simulink model "FPGA_MODELSIM"  (R2019b)
settings: Solver=ode1  StartTime=0.0  StopTime=1  FixedStep=1e-4  RelTol=1e-3
InitFcn:
  | Ts=1e-4
  | T=1e-5
values from neighbouring files (symbols this model uses):
  B = 0.0136    [Pmsm.m]
  J = 0.0027    [Pmsm.m]
  Kiq = double(Kiq)    [Pmsm.m]
  Kiw = double(Kiw)    [Pmsm.m]
  Kpq = double(Kpq)    [Pmsm.m]
  Kpw = double(Kpw)    [Pmsm.m]
  Lambda_m = 0.2026    [Pmsm.m]
  Ld = 19.75e-3    (= 0.01975)    [Pmsm.m]
  Lq = 22.5e-3    (= 0.0225)    [Pmsm.m]
  P = 8    [Pmsm.m]
  Rs = 1.477    [Pmsm.m]
libraries: modelsimlib x2
settings Model: Creator=samfi  LastModifiedBy=samfi

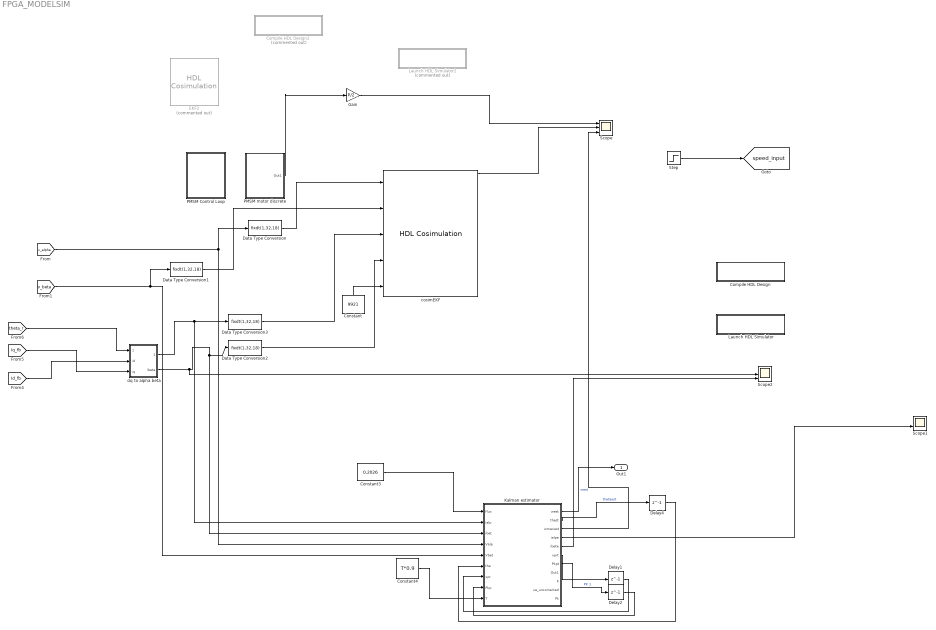
== system FPGA_MODELSIM ==
  Compile HDL Design : Subsystem
      settings: OpenFcn=eval('compile_hdl_design_cosimEKF');
      mask Display: disp(['Double-Click to' char(10) 'compile HDL files'])
  Compile HDL Design2 : Subsystem  Commented=on
      settings: OpenFcn=eval('compile_hdl_design_EKF');
      mask Display: disp(['Double-Click to' char(10) 'compile HDL files'])
  Constant : Constant  Value=9921  OutDataTypeStr=uint32  SampleTime=1e-4
  Constant3 : Constant  Value=0.2026
  Constant4 : Constant  Value=T*0.9  SampleTime=1e-4
  Data Type Conversion{,1..3} (4 alike) : DataTypeConversion  OutDataTypeStr=fixdt(1,32,18)
  Delay1 : Delay  DelayLength=1  InitialCondition=0
  Delay2 : Delay  DelayLength=1  InitialCondition=0
  Delay4 : Delay  DelayLength=1  InitialCondition=0
  EKF2 : modelsimlib/HDL Cosimulation  Commented=on  PortPaths=/EKF/valpha;/EKF/vbeta;/EKF/ialpham;/EKF/ibetam;/EKF/ctheta;/EKF/stheta;/EKF/nbSamples;/EKF/omega;/EKF/theta  PortModes=[1 1 1 1 1 1 1 2 2 ]  PortTimes=[-1,-1,-1,-1,-1,-1,-1,1e-4,1e-4]  PortSigns=[-1 -1 -1 -1 -1 -1 -1 1 1 ]  PortFracLengths=[0,0,0,0,0,0,0,18,18]  CommLocal=on  CommSharedMemory=on  CommPortNumber=4449  CommShowInfo=on  ClockModes=[]  ClockTimes=[]  TclPreSimCommand=|  TclPostSimCommand=|  TimingMode=s  TimingScaleFactor=1  idxCellArray={'UNUSED_VAR'}  CosimBypass=Full Simulation  AllowDirectFeedthrough=on  ProductName=EDA Simulator Link MQ  RunAutoTimescale=off  HdlClocks=/EKF/clk 10 ns;  PreRunTime=10  PreRunTimeUnit=ns
      TclPreSimCommand=|
      | force /EKF/clk 0 0 ns, 1 5 ns -repeat 10 ns;
      | force /EKF/reset 0 0 ns, 1 8 ns;
      TclPostSimCommand=|
      | noforce /EKF/clk;
      | noforce /EKF/reset;
      | puts "done";
      settings: SourceProductName=HDL Verifier  SourceProductBaseCode=ES
  Gain : Gain  Gain=P/2
  Kalman estimator : Subsystem  SystemSampleTime=1e-4
  Launch HDL Simulator : Subsystem
      settings: OpenFcn=eval('launch_hdl_simulator_cosimEKF');
      mask Display: disp(['Double-Click to' char(10) 'launch HDL simulator'])
  Launch HDL Simulator2 : Subsystem  Commented=on
      settings: OpenFcn=eval('launch_hdl_simulator_EKF');
      mask Display: disp(['Double-Click to' char(10) 'launch HDL simulator'])
  PMSM Control Loop : Subsystem
  PMSM motor discrete : Subsystem
  Scope : Scope  NumInputPorts=3
  Scope1 : Scope  NumInputPorts=2
  Scope2 : Scope  NumInputPorts=3
  Step : Step  Time=0  After=500  SampleTime=1e-4
  cosimEKF : modelsimlib/HDL Cosimulation  PortPaths=/cosimEKF/valpha;/cosimEKF/vbeta;/cosimEKF/ialpham;/cosimEKF/ibetam;/cosimEKF/nbSamples;/cosimEKF/omega;/cosimEKF/theta;/cosimEKF/ialphak;/cosimEKF/ibetak;/cosimEKF/kmatrix00;/cosimEKF/kmatrix01;/cosimEKF/kmatrix10;/cosimEKF/kmatrix11;/cosimEKF/kmatrix20;/cosimEKF/kmatrix21;/cosimEKF/kmatrix30;/cosimEKF/kmatrix31  PortModes=[1 1 1 1 1 2 2 2 2 2 2 2 2 2 2 2 2 ]  PortTimes=[-1,-1,-1,-1,-1,1e-4,1e-4,1,1,1,1,1,1,1,1,1,1]  PortSigns=[-1 -1 -1 -1 -1 1 1 1 1 1 1 1 1 1 1 1 1 ]  PortFracLengths=[0,0,0,0,0,18,18,18,18,18,18,18,18,18,18,18,18]  CommLocal=on  CommSharedMemory=off  CommPortNumber=58870  CommShowInfo=on  ClockModes=[]  ClockTimes=[]  TclPreSimCommand=|  TclPostSimCommand=|  TimingMode=s  TimingScaleFactor=1  idxCellArray={'UNUSED_VAR'}  CosimBypass=Full Simulation  AllowDirectFeedthrough=on  ProductName=EDA Simulator Link MQ  RunAutoTimescale=off  HdlClocks=/cosimEKF/clk 10 ns;  PreRunTime=10  PreRunTimeUnit=ns
      TclPreSimCommand=|
      | force /cosimEKF/clk 0 0 ns, 1 5 ns -repeat 10 ns;
      | force /cosimEKF/reset 0 0 ns, 1 8 ns;
      TclPostSimCommand=|
      | noforce /cosimEKF/clk;
      | noforce /cosimEKF/reset;
      | puts "done";
      settings: SourceProductName=HDL Verifier  SourceProductBaseCode=ES
  dq to alpha beta : Subsystem
  Out1 : Outport
  tag scope: speed_input=global
  wires:
  Data Type Conversion/1 -> cosimEKF/1
  [Iq_fb] -> dq to alpha beta/3(iq)
  dq to alpha beta/1(ialpha) -> Kalman estimator/2(ialp), Data Type Conversion3/1
  [theta_r] -> dq to alpha beta/1(theta_r)
  [Id_fb] -> dq to alpha beta/2(id)
  Constant/1 -> cosimEKF/5
  [v_alpha] -> Kalman estimator/4(Valp), Data Type Conversion/1
  Data Type Conversion1/1 -> cosimEKF/2
  Data Type Conversion2/1 -> cosimEKF/4
  Kalman estimator/7(Pkpt) -> Delay2/1  "PK 1"
  Kalman estimator/6(xprt) -> Delay1/1
  Delay2/1 -> Kalman estimator/8(Pkp)
  Delay1/1 -> Kalman estimator/7(xpr)
  Kalman estimator/3(wmecest) -> Scope/3
  Kalman estimator/1(west) -> Out1/1  "west"
  Kalman estimator/2(thest) -> Delay4/1  "thetaest"
  Constant3/1 -> Kalman estimator/1(flux)
  Constant4/1 -> Kalman estimator/9(T)
  Delay4/1 -> Kalman estimator/6(the)
  Step/1 -> [speed_input]
  PMSM motor discrete/1(Out1) -> Gain/1
  Kalman estimator/4(ialpe) -> Scope1/2
  Kalman estimator/5(ibete) -> Scope2/3
  dq to alpha beta/2(ibeta) -> Scope2/2, Kalman estimator/3(ibet), Data Type Conversion2/1
  [v_beta] -> Kalman estimator/5(Vbet), Data Type Conversion1/1
  Data Type Conversion3/1 -> cosimEKF/3
  Gain/1 -> Scope/1
  cosimEKF/1 -> Scope/2

== system FPGA_MODELSIM/Compile HDL Design ==

== system FPGA_MODELSIM/Compile HDL Design2 ==

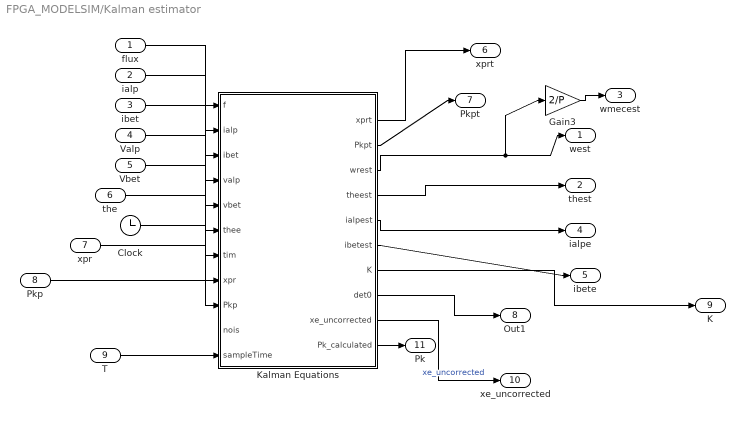
== system FPGA_MODELSIM/Kalman estimator ==
  flux : Inport
  ialp : Inport  Port=2
  ibet : Inport  Port=3
  Valp : Inport  Port=4
  Vbet : Inport  Port=5
  the : Inport  Port=6
  xpr : Inport  Port=7
  Pkp : Inport  Port=8
  T : Inport  Port=9
  Clock : Clock
  Gain3 : Gain  Gain=2/P
  Kalman Equations : MATLAB Function  TreatAsAtomicUnit=on  SystemSampleTime=1e-4
  west : Outport
  thest : Outport  Port=2
  wmecest : Outport  Port=3
  ialpe : Outport  Port=4
  ibete : Outport  Port=5
  xprt : Outport  Port=6
  Pkpt : Outport  Port=7
  Out1 : Outport  Port=8
  K : Outport  Port=9
  "xe_uncorrected " : Outport  Port=10
  Pk : Outport  Port=11
  wires:
  T/1 -> Kalman Equations/11(sampleTime)
  Pkp/1 -> Kalman Equations/9(Pkp)
  xpr/1 -> Kalman Equations/8(xpr)
  the/1 -> Kalman Equations/6(thee)
  Kalman Equations/2(Pkpt) -> Pkpt/1
  Kalman Equations/1(xprt) -> xprt/1
  Kalman Equations/6(ibetest) -> ibete/1
  Kalman Equations/5(ialpest) -> ialpe/1
  ibet/1 -> Kalman Equations/3(ibet)
  ialp/1 -> Kalman Equations/2(ialp)
  Gain3/1 -> wmecest/1
  Kalman Equations/4(theest) -> thest/1
  Kalman Equations/3(wrest) -> Gain3/1, west/1
  Clock/1 -> Kalman Equations/7(tim)
  Vbet/1 -> Kalman Equations/5(vbet)
  Valp/1 -> Kalman Equations/4(valp)
  flux/1 -> Kalman Equations/1(f)
  Kalman Equations/8(det0) -> Out1/1
  Kalman Equations/7(K) -> K/1
  Kalman Equations/9(xe_uncorrected) -> "xe_uncorrected "/1  "xe_uncorrected"
  Kalman Equations/10(Pk_calculated) -> Pk/1

== system FPGA_MODELSIM/Launch HDL Simulator ==

== system FPGA_MODELSIM/Launch HDL Simulator2 ==

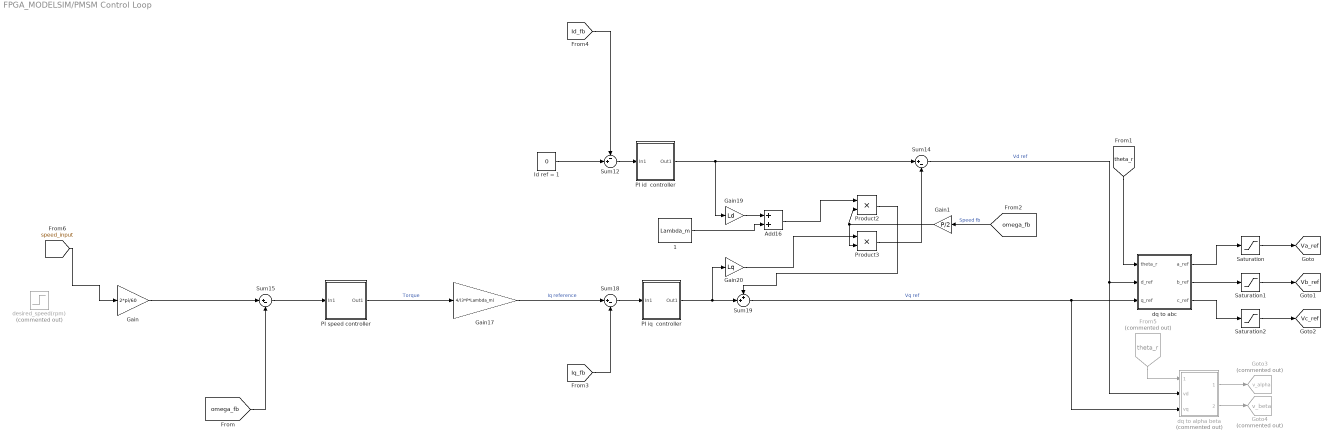
== system FPGA_MODELSIM/PMSM Control Loop ==
  " 1" : Constant  Value=Lambda_m
  Add16 : Sum
  From5 : From  Commented=on  GotoTag=theta_r  TagVisibility=global
  Gain : Gain  Gain=2*pi/60
  Gain1 : Gain  Gain=P/2
  Gain17 : Gain  Gain=4/(3*P*Lambda_m)
  Gain19 : Gain  Gain=Ld
  Gain20 : Gain  Gain=Lq
  Goto3 : Goto  Commented=on  GotoTag=v_alpha  TagVisibility=global
  Goto4 : Goto  Commented=on  GotoTag=v_beta  TagVisibility=global
  Id ref = 1 : Constant  Value=0  SampleTime=Ts
  PI id  controller : Subsystem
  PI iq  controller : Subsystem
  PI speed controller : Subsystem
  Product2 : Product
  Product3 : Product
  Saturation : Saturate  UpperLimit=220  LowerLimit=-220
  Saturation1 : Saturate  UpperLimit=200  LowerLimit=-200
  Saturation2 : Saturate  UpperLimit=200  LowerLimit=-200
  Sum12 : Sum  Inputs=-+|
  Sum14 : Sum  Inputs=|+-
  Sum15 : Sum  Inputs=|+-
  Sum18 : Sum  Inputs=|+-
  Sum19 : Sum  Inputs=++|
  desired_speed(rpm) : Step  Commented=on  Time=0.25  After=500  SampleTime=0
  dq to abc : Subsystem
  dq to alpha beta : Subsystem  Commented=on
  tag scope: Va_ref=global, Vb_ref=global, Vc_ref=global
  wires:
  Product2/1 -> Sum19/1
  Add16/1 -> Product2/1
  Gain20/1 -> Product3/1
  Product3/1 -> Sum14/2
  Id ref = 1/1 -> Sum12/2
  PI iq  controller/1(Out1) -> Gain20/1, Sum19/2
  PI id  controller/1(Out1) -> Gain19/1, Sum14/1
  Sum14/1 -> dq to alpha beta/2(vd), dq to abc/2(d_ref)  "Vd ref"
  Gain19/1 -> Add16/1
  Sum18/1 -> PI iq  controller/1(In1)
  " 1"/1 -> Add16/2
  Gain17/1 -> Sum18/1  "Iq reference"
  Sum19/1 -> dq to alpha beta/3(vq), dq to abc/3(q_ref)  "Vq ref"
  [omega_fb] -> Sum15/2
  [theta_r] -> dq to abc/1(theta_r)
  [Iq_fb] -> Sum18/2
  [Id_fb] -> Sum12/1
  Saturation/1 -> [Va_ref]
  Saturation1/1 -> [Vb_ref]
  Saturation2/1 -> [Vc_ref]
  dq to abc/3(c_ref) -> Saturation2/1
  dq to abc/1(a_ref) -> Saturation/1
  dq to abc/2(b_ref) -> Saturation1/1
  Gain/1 -> Sum15/1
  [omega_fb] -> Gain1/1  "Speed fb"
  Gain1/1 -> Product3/2, Product2/2
  Sum12/1 -> PI id  controller/1(In1)
  Sum15/1 -> PI speed controller/1(In1)
  PI speed controller/1(Out1) -> Gain17/1  "Torque"
  dq to alpha beta/1(valpha) -> Goto3/1
  dq to alpha beta/2(vbeta) -> Goto4/1
  From5/1 -> dq to alpha beta/1(theta_r)
  [speed_input] -> Gain/1

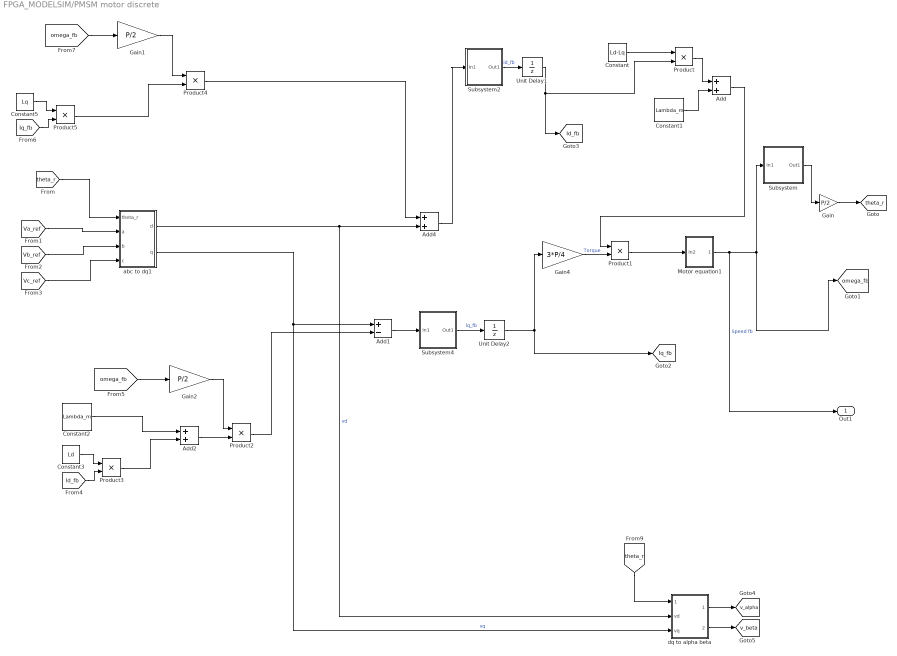
== system FPGA_MODELSIM/PMSM motor discrete ==
  Add : Sum
  Add1 : Sum  Inputs=+-
  Add2 : Sum
  Add4 : Sum
  Constant : Constant  Value=Ld-Lq  SampleTime=Ts
  Constant1 : Constant  Value=Lambda_m
  Constant2 : Constant  Value=Lambda_m
  Constant3 : Constant  Value=Ld  SampleTime=Ts
  Constant5 : Constant  Value=Lq  SampleTime=Ts
  Gain : Gain  Gain=P/2
  Gain1 : Gain  Gain=P/2
  Gain2 : Gain  Gain=P/2
  Gain4 : Gain  Gain=3*P/4
  Motor equation1 : Subsystem
  Product{,1..5} (6 alike) : Product
  Subsystem : Subsystem
  Subsystem2 : Subsystem
  Subsystem4 : Subsystem
  Unit Delay1 : UnitDelay  SampleTime=-1  HasFrameUpgradeWarning=on
  Unit Delay2 : UnitDelay  SampleTime=-1  HasFrameUpgradeWarning=on
  abc to dq1 : Subsystem
  dq to alpha beta : Subsystem
  Out1 : Outport
  tag scope: Id_fb=global, Iq_fb=global, omega_fb=global, theta_r=global, v_alpha=global, v_beta=global
  wires:
  Subsystem4/1(Out1) -> Unit Delay2/1  "iq_fb"
  [Vb_ref] -> abc to dq1/3(b)
  Motor equation1/1(Out1) -> Out1/1, [omega_fb], Subsystem/1(In1)  "Speed fb"
  [Va_ref] -> abc to dq1/2(a)
  [Vc_ref] -> abc to dq1/4(c)
  Subsystem2/1(Out1) -> Unit Delay1/1  "id_fb"
  Product1/1 -> Motor equation1/1(In2)
  Constant/1 -> Product/1
  Product/1 -> Add/1
  Constant1/1 -> Add/2
  Gain4/1 -> Product1/2  "Torque"
  Add/1 -> Product1/1
  Subsystem/1(Out1) -> Gain/1
  Gain/1 -> [theta_r]
  abc to dq1/2(q) -> dq to alpha beta/3(vq), Add1/1  "vq"
  Product2/1 -> Add1/2
  [omega_fb] -> Gain2/1
  Constant3/1 -> Product3/1
  [Id_fb] -> Product3/2
  Product3/1 -> Add2/2
  Constant2/1 -> Add2/1
  Add2/1 -> Product2/2
  [Iq_fb] -> Product5/2
  Product5/1 -> Product4/2
  Constant5/1 -> Product5/1
  abc to dq1/1(d) -> dq to alpha beta/2(vd), Add4/2  "vd"
  Product4/1 -> Add4/1
  [omega_fb] -> Gain1/1
  Gain1/1 -> Product4/1
  Gain2/1 -> Product2/1
  dq to alpha beta/1(valpha) -> [v_alpha]
  dq to alpha beta/2(vbeta) -> [v_beta]
  [theta_r] -> abc to dq1/1(theta_r)
  [theta_r] -> dq to alpha beta/1(theta_r)
  Add4/1 -> Subsystem2/1(In1)
  Add1/1 -> Subsystem4/1(In1)
  Unit Delay1/1 -> [Id_fb], Product/2
  Unit Delay2/1 -> Gain4/1, [Iq_fb]

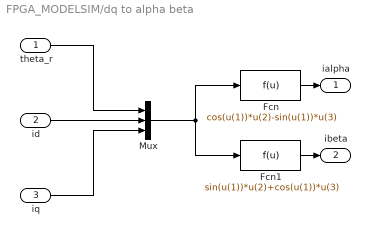
== system FPGA_MODELSIM/dq to alpha beta ==
  theta_r : Inport
  id : Inport  Port=2
  iq : Inport  Port=3
  Fcn : Fcn  Expr=cos(u(1))*u(2)-sin(u(1))*u(3)
  Fcn1 : Fcn  Expr=sin(u(1))*u(2)+cos(u(1))*u(3)
  Mux : Mux  Inputs=3
  ialpha : Outport
  ibeta : Outport  Port=2
  wires:
  Mux/1 -> Fcn/1, Fcn1/1
  iq/1 -> Mux/3
  theta_r/1 -> Mux/1
  Fcn1/1 -> ibeta/1
  id/1 -> Mux/2
  Fcn/1 -> ialpha/1

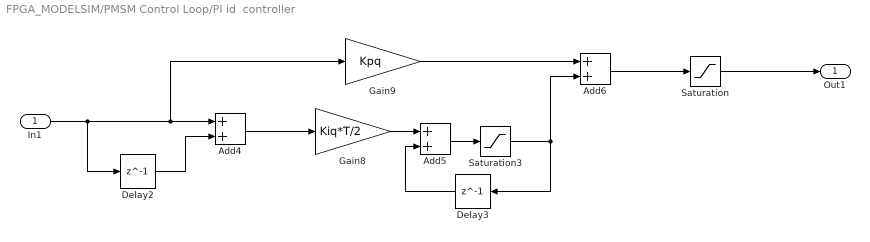
== system FPGA_MODELSIM/PMSM Control Loop/PI id  controller ==
  In1 : Inport
  Add4 : Sum
  Add5 : Sum
  Add6 : Sum
  Delay2 : Delay  DelayLength=1
  Delay3 : Delay  DelayLength=1
  Gain8 : Gain  Gain=Kiq*T/2
  Gain9 : Gain  Gain=Kpq
  Saturation : Saturate  UpperLimit=220  LowerLimit=-220
  Saturation3 : Saturate  UpperLimit=200  LowerLimit=-200
  Out1 : Outport
  wires:
  Gain8/1 -> Add5/1
  Delay2/1 -> Add4/2
  Add5/1 -> Saturation3/1
  Add4/1 -> Gain8/1
  Saturation3/1 -> Delay3/1, Add6/2
  In1/1 -> Add4/1, Gain9/1, Delay2/1
  Gain9/1 -> Add6/1
  Delay3/1 -> Add5/2
  Add6/1 -> Saturation/1
  Saturation/1 -> Out1/1

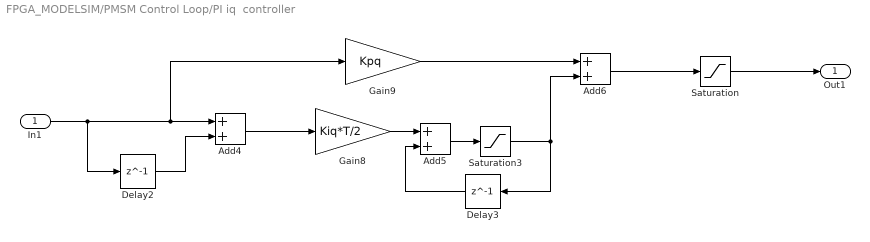
== system FPGA_MODELSIM/PMSM Control Loop/PI iq  controller ==
  In1 : Inport
  Add4 : Sum
  Add5 : Sum
  Add6 : Sum
  Delay2 : Delay  DelayLength=1
  Delay3 : Delay  DelayLength=1
  Gain8 : Gain  Gain=Kiq*T/2
  Gain9 : Gain  Gain=Kpq
  Saturation : Saturate  UpperLimit=220  LowerLimit=-220
  Saturation3 : Saturate  UpperLimit=200  LowerLimit=-200
  Out1 : Outport
  wires:
  Delay3/1 -> Add5/2
  Gain9/1 -> Add6/1
  In1/1 -> Delay2/1, Gain9/1, Add4/1
  Saturation3/1 -> Add6/2, Delay3/1
  Add4/1 -> Gain8/1
  Add5/1 -> Saturation3/1
  Delay2/1 -> Add4/2
  Gain8/1 -> Add5/1
  Add6/1 -> Saturation/1
  Saturation/1 -> Out1/1

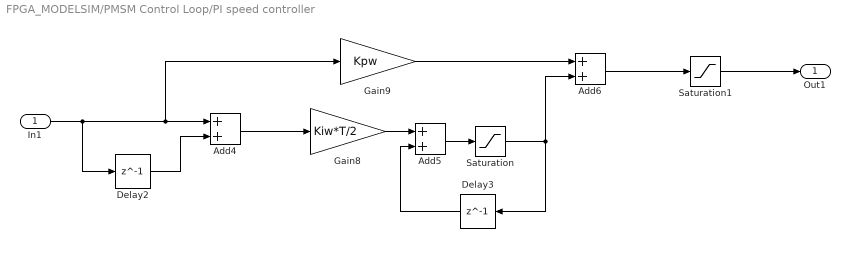
== system FPGA_MODELSIM/PMSM Control Loop/PI speed controller ==
  In1 : Inport
  Add4 : Sum
  Add5 : Sum
  Add6 : Sum
  Delay2 : Delay  DelayLength=1
  Delay3 : Delay  DelayLength=1
  Gain8 : Gain  Gain=Kiw*T/2
  Gain9 : Gain  Gain=Kpw
  Saturation : Saturate  UpperLimit=10  LowerLimit=-10
  Saturation1 : Saturate  UpperLimit=10  LowerLimit=-10
  Out1 : Outport
  wires:
  Gain9/1 -> Add6/1
  Delay2/1 -> Add4/2
  Gain8/1 -> Add5/1
  Add5/1 -> Saturation/1
  In1/1 -> Delay2/1, Gain9/1, Add4/1
  Saturation/1 -> Add6/2, Delay3/1
  Add4/1 -> Gain8/1
  Delay3/1 -> Add5/2
  Add6/1 -> Saturation1/1
  Saturation1/1 -> Out1/1

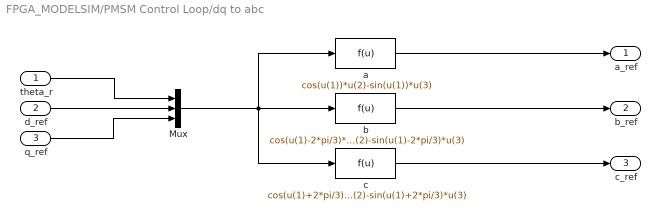
== system FPGA_MODELSIM/PMSM Control Loop/dq to abc ==
  theta_r : Inport
  d_ref : Inport  Port=2
  q_ref : Inport  Port=3
  Mux : Mux  Inputs=3
  a : Fcn  Expr=cos(u(1))*u(2)-sin(u(1))*u(3)
  b : Fcn  Expr=cos(u(1)-2*pi/3)*u(2)-sin(u(1)-2*pi/3)*u(3)
  c : Fcn  Expr=cos(u(1)+2*pi/3)*u(2)-sin(u(1)+2*pi/3)*u(3)
  a_ref : Outport
  b_ref : Outport  Port=2
  c_ref : Outport  Port=3
  wires:
  d_ref/1 -> Mux/2
  Mux/1 -> c/1, b/1, a/1
  c/1 -> c_ref/1
  theta_r/1 -> Mux/1
  b/1 -> b_ref/1
  a/1 -> a_ref/1
  q_ref/1 -> Mux/3

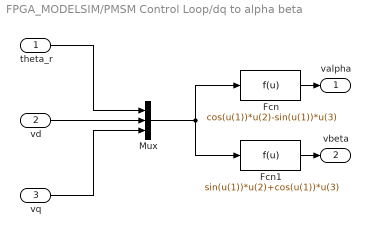
== system FPGA_MODELSIM/PMSM Control Loop/dq to alpha beta ==
  theta_r : Inport
  vd : Inport  Port=2
  vq : Inport  Port=3
  Fcn : Fcn  Expr=cos(u(1))*u(2)-sin(u(1))*u(3)
  Fcn1 : Fcn  Expr=sin(u(1))*u(2)+cos(u(1))*u(3)
  Mux : Mux  Inputs=3
  valpha : Outport
  vbeta : Outport  Port=2
  wires:
  Mux/1 -> Fcn/1, Fcn1/1
  vq/1 -> Mux/3
  theta_r/1 -> Mux/1
  Fcn1/1 -> vbeta/1
  vd/1 -> Mux/2
  Fcn/1 -> valpha/1

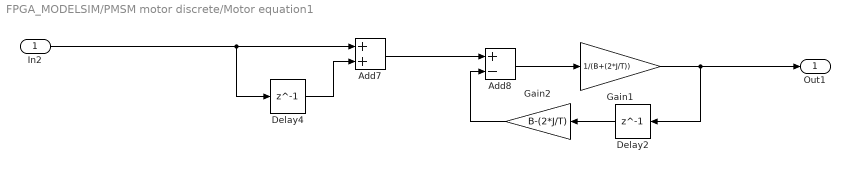
== system FPGA_MODELSIM/PMSM motor discrete/Motor equation1 ==
  In2 : Inport
  Add7 : Sum
  Add8 : Sum  Inputs=+-
  Delay2 : Delay  DelayLength=1
  Delay4 : Delay  DelayLength=1
  Gain1 : Gain  Gain=1/(B+(2*J/T))
  Gain2 : Gain  Gain=B-(2*J/T)
  Out1 : Outport
  wires:
  Add7/1 -> Add8/1
  Gain1/1 -> Out1/1, Delay2/1
  Delay2/1 -> Gain2/1
  Add8/1 -> Gain1/1
  Gain2/1 -> Add8/2
  In2/1 -> Delay4/1, Add7/1
  Delay4/1 -> Add7/2

== system FPGA_MODELSIM/PMSM motor discrete/Subsystem ==
  In1 : Inport
  Add1 : Sum
  Add2 : Sum
  Delay1 : Delay  DelayLength=1
  Delay4 : Delay  DelayLength=1
  Gain : Gain  Gain=T/2
  Out1 : Outport
  wires:
  In1/1 -> Delay4/1, Add1/1
  Delay1/1 -> Add2/2
  Add2/1 -> Out1/1, Delay1/1
  Delay4/1 -> Add1/2
  Add1/1 -> Gain/1
  Gain/1 -> Add2/1

== system FPGA_MODELSIM/PMSM motor discrete/Subsystem2 ==
  In1 : Inport
  Add7 : Sum
  Add8 : Sum  Inputs=+-
  Delay2 : Delay  DelayLength=1
  Delay4 : Delay  DelayLength=1
  Gain1 : Gain  Gain=1/(Rs+(2*Ld/T))
  Gain2 : Gain  Gain=Rs-(2*Ld/T)
  Out1 : Outport
  wires:
  Add8/1 -> Gain1/1
  In1/1 -> Add7/1, Delay4/1
  Gain2/1 -> Add8/2
  Delay2/1 -> Gain2/1
  Delay4/1 -> Add7/2
  Add7/1 -> Add8/1
  Gain1/1 -> Out1/1, Delay2/1

== system FPGA_MODELSIM/PMSM motor discrete/Subsystem4 ==
  In1 : Inport
  Add7 : Sum
  Add8 : Sum  Inputs=+-
  Delay2 : Delay  DelayLength=1
  Delay4 : Delay  DelayLength=1
  Gain1 : Gain  Gain=1/(Rs+(2*Lq/T))
  Gain2 : Gain  Gain=Rs-(2*Lq/T)
  Out1 : Outport
  wires:
  Add8/1 -> Gain1/1
  Gain1/1 -> Delay2/1, Out1/1
  Add7/1 -> Add8/1
  Delay4/1 -> Add7/2
  Delay2/1 -> Gain2/1
  Gain2/1 -> Add8/2
  In1/1 -> Delay4/1, Add7/1

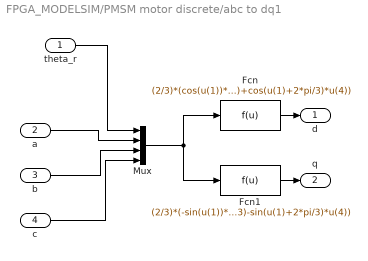
== system FPGA_MODELSIM/PMSM motor discrete/abc to dq1 ==
  theta_r : Inport
  a : Inport  Port=2
  b : Inport  Port=3
  c : Inport  Port=4
  Fcn : Fcn  Expr=(2/3)*(cos(u(1))*u(2)+cos(u(1)-2*pi/3)*u(3)+cos(u(1)+2*pi/3)*u(4))
  Fcn1 : Fcn  Expr=(2/3)*(-sin(u(1))*u(2)-sin(u(1)-2*pi/3)*u(3)-sin(u(1)+2*pi/3)*u(4))
  Mux : Mux
  d : Outport
  q : Outport  Port=2
  wires:
  a/1 -> Mux/2
  c/1 -> Mux/4
  theta_r/1 -> Mux/1
  Mux/1 -> Fcn/1, Fcn1/1
  b/1 -> Mux/3
  Fcn/1 -> d/1
  Fcn1/1 -> q/1

== system FPGA_MODELSIM/PMSM motor discrete/dq to alpha beta ==
  theta_r : Inport
  vd : Inport  Port=2
  vq : Inport  Port=3
  Fcn : Fcn  Expr=cos(u(1))*u(2)-sin(u(1))*u(3)
  Fcn1 : Fcn  Expr=sin(u(1))*u(2)+cos(u(1))*u(3)
  Mux : Mux  Inputs=3
  valpha : Outport
  vbeta : Outport  Port=2
  wires:
  Mux/1 -> Fcn/1, Fcn1/1
  vq/1 -> Mux/3
  theta_r/1 -> Mux/1
  Fcn1/1 -> vbeta/1
  vd/1 -> Mux/2
  Fcn/1 -> valpha/1

== matlab function FPGA_MODELSIM/Kalman estimator/Kalman Equations ==
  data: f input; xprt output; ialp input; ibet input; valp input; vbet input; thee input; tim input; Pkpt output; xpr input; Pkp input; wrest output; theest output; ialpest output; ibetest output; nois input; sampleTime input; K output; det0 output; xe_uncorrected output; Pk_calculated output
function [xprt,Pkpt,wrest,theest,ialpest,ibetest,K,det0,xe_uncorrected,Pk_calculated]     = fcn(f,ialp,ibet,valp,vbet,thee,tim,xpr,Pkp,nois,sampleTime)
%#eml

% xprt=[0;0;0;0];
%     Pkpt=[0.1 0 0 0;0 0.1 0 0;0 0 0.1 0;0 0 0 0.1];
if tim==0
    xprt=[0;0;0;0];
    xe_uncorrected=[0;0;0;0];
    tim;
    Pkpt=[5 0 0 0;0 5 0 0;0 0 10 0;0 0 0 1];
    Pk_calculated = [0 0 0 0;
                        0 0 0 0;
                        0 0 0 0;
                        0 0 0 0];
    wrest=0;
    theest=0;
    thee=0;
    ialpest=0;
    ibetest=0;
    wef=0;
    K=[0 0; 0 0; 0 0; 0 0];
    det0 = 0;
    thrq=0;
end

%Q=.085,.085, 15.2,0 gives same as .01,.01,5.2,0 same as .2,.2.45.2,0
Q=[0.01 0 0 0;0 0.01 0 0;0 0 50 0;0 0 0 0.0001];


J = 0.0027;
B = 0.0136;
r=1.477;
Ld=19.75e-3;
p=8;
Lq=22.5e-3;
Ts=sampleTime;
L1=(Ld+Lq)/2;
L2=(Ld-Lq)/2;

%Tef=(3*p/4)*(f*iqest+(Ld-Lq)*idest*iqest);
ial=xpr(1,1);
ibe=xpr(2,1);
we=xpr(3,1);
thee=xpr(4,1);


I=[1 0 0 0;0 1 0 0;0 0 1 0;0 0 0 1];

xe=[ial+((valp/L1)-(r*ial/L1)+(we*f*sin(thee)/L1))*Ts;
    ibe+((vbet/L1)-(r*ibe/L1)-(we*f*cos(thee)/L1))*Ts;
    we;
    thee+(we*Ts)];

F=[1-(r*Ts/L1) 0 (Ts*f*sin(thee))/L1 (we*f*cos(thee)*Ts)/L1;
    0 1-(r*Ts/L1) -(Ts*f*cos(thee))/L1 (we*f*sin(thee)*Ts)/L1;
    0 0 1 0;
    0 0 Ts 1];%
% G=[1-(Ts/taud) Ts*xpr(3,1)*Lq/Ld Ts*Lq*xe(2,1)/Ld 0;
%     -Ld*Ts*xpr(3,1)/Lq 1-(Ts/tauq) Ts*(((-Ld/Lq)*xe(1,1))-(f/Lq)) 0;
%     (3*p/4)*((Ld-Lq)*xpr(2,1))*Ts (3*p/4)*(f+(Ld-Lq)*xpr(1,1))*Ts 1-((B/J)*Ts) 0;
%     0 0 Ts 1];

% end
Rd=0.92;
R=[Rd 0;0 Rd];
%noise=sqrt(Rd/7)*randn;
yk=[ialp;ibet];%+[noise;noise];
C=[1 0 0 0;
    0 1 0 0];
Pk=F*Pkp*transpose(F)+Q;
Pk_calculated = Pk;
K=Pk*transpose(C)/(C*Pk*transpose(C)+R);
x=xe+K*(yk-C*xe);
P=(I-K*C)*Pk;
det0 = det(C*Pk*transpose(C)+R);
xprt=I*x;
Pkpt=I*P;
wrest=x(3,1);
theest=x(4,1);
ialpest=x(1,1);
ibetest=x(2,1);
xe_uncorrected = xe;
end
